simulink model "lab4_simulink"  (R2022b)
settings: Solver=VariableStepAuto  StartTime=0.0  StopTime=czas_symulacji  RelTol=1e-3
values from neighbouring files (symbols this model uses):
  Cvp = cp*rop*Vp    (= 36000)    [lab4_przygotowanie.m]
  Cvw = cp*rop*Vw    (= 67200)    [lab4_przygotowanie.m]
  dqg = 0.1*qgN    (= 1000)    [lab4_przygotowanie.m]
  dTzew = 1    [lab4_przygotowanie.m]
  kcp = (z*qgN*(TwewN-TpN))/((TpN-TzewN)*((TwewN-TzewN)+z*(TwewN-TpN)))    (= 23.2558139535)    [lab4_przygotowanie.m]
  kcw = qgN/(TwewN-TzewN+z*(TwewN-TpN))    (= 232.558139535)    [lab4_przygotowanie.m]
  kcwp = z*kcw    (= 69.7674418605)    [lab4_przygotowanie.m]
  qg0 = qgN*procent_zmiany_qg    (= 8000)    [lab4_przygotowanie.m]
  t0 = 1000    [lab4_przygotowanie.m]
  Tp0 = ((kcp*Tzew0)*(kcw+kcwp)+kcwp*(qg0+kcw*Tzew0))/(kcwp*kcw+kcp*kcw+kcp*kcwp)    [lab4_przygotowanie.m]
  Twew0 = (qg0+kcw*Tzew0+kcwp*Tp0)/(kcw+kcwp)    [lab4_przygotowanie.m]
  Tzew0 = TzewN+zmianaTzew(i)    [lab4_przygotowanie.m]
settings Model: Creator=Dawid  LastModifiedBy=Dawid
settings DataIOCC: ReturnWorkspaceOutputs=off

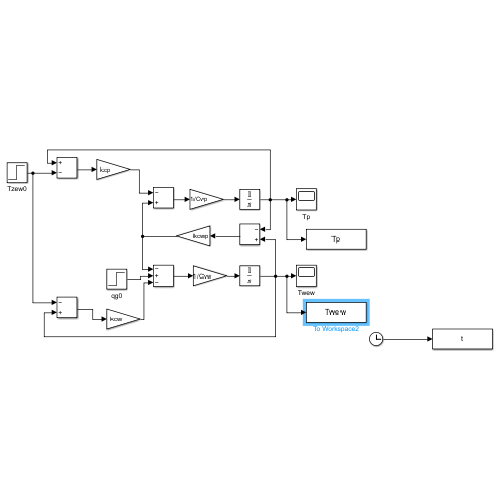
[thumbnail: Simulink's stored preview of the top-level diagram]
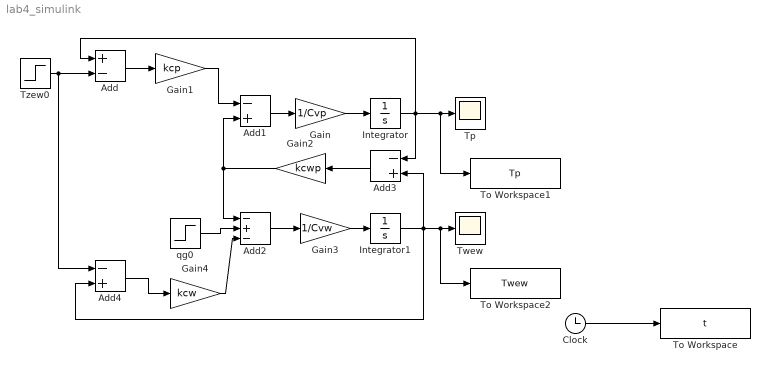
== system lab4_simulink ==
  Add : Sum  Inputs=+-
  Add1 : Sum  Inputs=-+
  Add2 : Sum  Inputs=-+-
  Add3 : Sum  Inputs=-+
  Add4 : Sum  Inputs=-+
  Clock : Clock
  Gain : Gain  Gain=1/Cvp
  Gain1 : Gain  Gain=kcp
  Gain2 : Gain  Gain=kcwp
  Gain3 : Gain  Gain=1/Cvw
  Gain4 : Gain  Gain=kcw
  Integrator : Integrator  InitialCondition=Tp0
  Integrator1 : Integrator  InitialCondition=Twew0
  To Workspace : ToWorkspace  VariableName=t  SaveFormat=Timeseries  SampleTime=-1
  To Workspace1 : ToWorkspace  VariableName=Tp  SampleTime=-1
  To Workspace2 : ToWorkspace  VariableName=Twew  SampleTime=-1
  Tp : Scope
  Twew : Scope
  Tzew0 : Step  Time=t0  Before=Tzew0  After=Tzew0+dTzew  SampleTime=0
  qg0 : Step  Time=t0  Before=qg0  After=qg0+dqg  SampleTime=0
  wires:
  Gain/1 -> Integrator/1
  Add1/1 -> Gain/1
  Add/1 -> Gain1/1
  Gain1/1 -> Add1/1
  qg0/1 -> Add2/2
  Gain2/1 -> Add1/2, Add2/1
  Add2/1 -> Gain3/1
  Gain3/1 -> Integrator1/1
  Add3/1 -> Gain2/1
  Integrator1/1 -> Add4/2, Add3/2, To Workspace2/1, Twew/1
  Integrator/1 -> To Workspace1/1, Tp/1, Add/1, Add3/1
  Clock/1 -> To Workspace/1
  Tzew0/1 -> Add/2, Add4/1
  Gain4/1 -> Add2/3
  Add4/1 -> Gain4/1
